simulink model "memory_matrix_test_tmp"  (Simulink 8.3)
settings: Solver=ode45  StartTime=0.0  StopTime=10.0  RelTol=1e-3
settings Model: Creator=arnaud  LastModifiedBy=hbourbou
settings DataIOCC: SaveFormat=Structure
settings OptimizationCC: ExpressionDepthLimit=2147483647
settings DebuggingCC: FcnCallInpInsideContextMsg=EnableAllAsWarning  FrameProcessingCompatibilityMsg=error

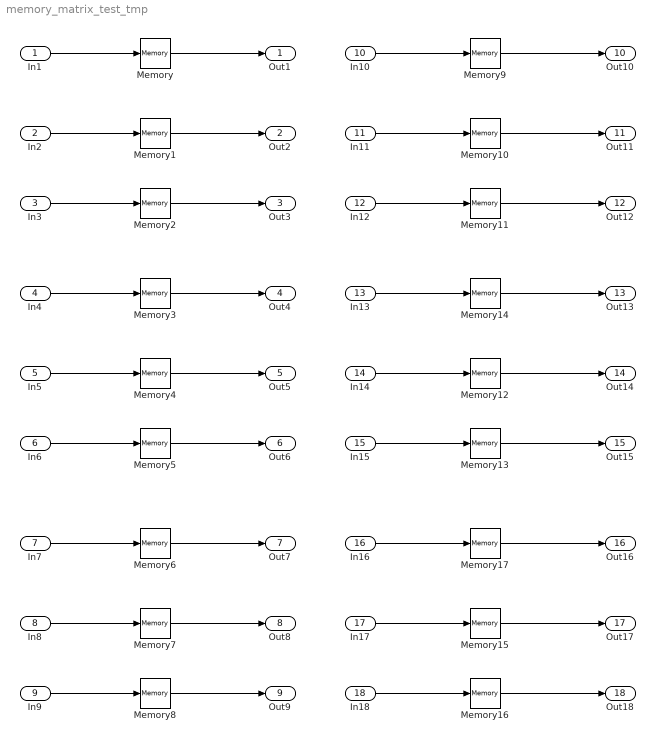
== system memory_matrix_test_tmp ==
  In1 : Inport  OutDataTypeStr=double  PortDimensions=[2 3]
  In2 : Inport  Port=2  OutDataTypeStr=double  PortDimensions=[2 3]
  In3 : Inport  Port=3  PortDimensions=[2 3]
  In4 : Inport  Port=4  OutDataTypeStr=int8  PortDimensions=[2 3]
  In5 : Inport  Port=5  OutDataTypeStr=int8  PortDimensions=[2 3]
  In6 : Inport  Port=6  OutDataTypeStr=int8  PortDimensions=[2 3]
  In7 : Inport  Port=7  OutDataTypeStr=boolean  PortDimensions=[2 3]
  In8 : Inport  Port=8  OutDataTypeStr=boolean  PortDimensions=[2 3]
  In9 : Inport  Port=9  OutDataTypeStr=boolean  PortDimensions=[2 3]
  In10 : Inport  Port=10  OutDataTypeStr=double  PortDimensions=[2 3]
  In11 : Inport  Port=11  OutDataTypeStr=double  PortDimensions=[2 3]
  In12 : Inport  Port=12  PortDimensions=[2 3]
  In13 : Inport  Port=13  OutDataTypeStr=int8  PortDimensions=[2 3]
  In14 : Inport  Port=14  OutDataTypeStr=int8  PortDimensions=[2 3]
  In15 : Inport  Port=15  OutDataTypeStr=int8  PortDimensions=[2 3]
  In16 : Inport  Port=16  OutDataTypeStr=boolean  PortDimensions=[2 3]
  In17 : Inport  Port=17  OutDataTypeStr=boolean  PortDimensions=[2 3]
  In18 : Inport  Port=18  OutDataTypeStr=boolean  PortDimensions=[2 3]
  Memory : Memory
  Memory1 : Memory  X0=0.0
  Memory{9..10,12,14..15,17} (6 alike) : Memory  X0=[0 2 3;4 5 6]
  Memory11 : Memory  X0=[true false true; false false false]
  Memory13 : Memory  X0=[true false true; false false false]
  Memory16 : Memory  X0=[true false true; false false false]
  Memory2 : Memory  X0=true
  Memory3 : Memory
  Memory4 : Memory  X0=0.0
  Memory5 : Memory  X0=true
  Memory6 : Memory
  Memory7 : Memory  X0=0.0
  Memory8 : Memory  X0=true
  Out1 : Outport
  Out2 : Outport  Port=2
  Out3 : Outport  Port=3
  Out4 : Outport  Port=4
  Out5 : Outport  Port=5
  Out6 : Outport  Port=6
  Out7 : Outport  Port=7
  Out8 : Outport  Port=8
  Out9 : Outport  Port=9
  Out10 : Outport  Port=10
  Out11 : Outport  Port=11
  Out12 : Outport  Port=12
  Out13 : Outport  Port=13
  Out14 : Outport  Port=14
  Out15 : Outport  Port=15
  Out16 : Outport  Port=16
  Out17 : Outport  Port=17
  Out18 : Outport  Port=18
  wires:
  In1/1 -> Memory/1
  Memory/1 -> Out1/1
  In2/1 -> Memory1/1
  Memory1/1 -> Out2/1
  In3/1 -> Memory2/1
  Memory2/1 -> Out3/1
  In4/1 -> Memory3/1
  Memory3/1 -> Out4/1
  In5/1 -> Memory4/1
  Memory4/1 -> Out5/1
  In6/1 -> Memory5/1
  Memory5/1 -> Out6/1
  In7/1 -> Memory6/1
  Memory6/1 -> Out7/1
  In8/1 -> Memory7/1
  Memory7/1 -> Out8/1
  In9/1 -> Memory8/1
  Memory8/1 -> Out9/1
  In10/1 -> Memory9/1
  Memory9/1 -> Out10/1
  In11/1 -> Memory10/1
  Memory10/1 -> Out11/1
  In12/1 -> Memory11/1
  Memory11/1 -> Out12/1
  In13/1 -> Memory14/1
  Memory14/1 -> Out13/1
  In14/1 -> Memory12/1
  Memory12/1 -> Out14/1
  In15/1 -> Memory13/1
  Memory13/1 -> Out15/1
  In16/1 -> Memory17/1
  Memory17/1 -> Out16/1
  In17/1 -> Memory15/1
  Memory15/1 -> Out17/1
  In18/1 -> Memory16/1
  Memory16/1 -> Out18/1
